simulink model "warp_timer"  (Simulink 7.1)
settings: Solver=ode45  StartTime=0.0  StopTime=1000  RelTol=1e-3
undefined symbols (not defined in the file): gcbh, xlBlockLoadCallback, xlGetSimulinkPeriod
libraries: xbsIndex_r4 x450
(part 1 of 5)
settings Model: Creator=CMC  LastModifiedBy=murphpo
settings DebuggingCC: SaveWithParameterizedLinksMsg=none  SignalResolutionControl=TryResolveAllWithWarning  MultiTaskDSMMsg=warning  MultiTaskCondExecSysMsg=none
settings RTWCC: IncludeERTFirstTime=on
settings GRTTargetCC: TargetFcnLib=ansi_tfl_tmw.mat

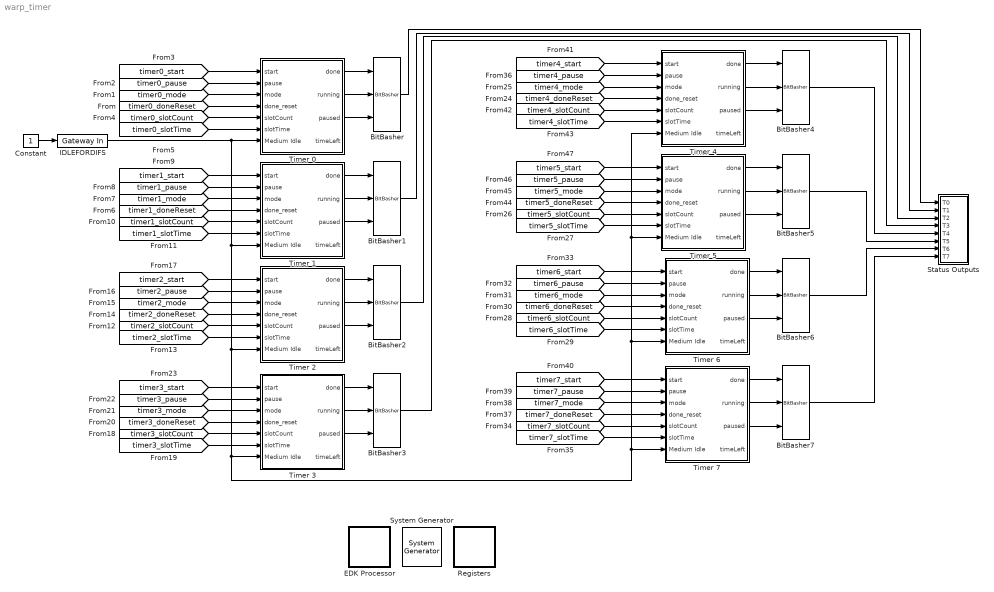
== system warp_timer ==
  " System Generator" : xbsIndex_r4/ System Generator  Tag=genX  SystemSampleTime=-1  xilinxfamily=virtex2p  part=xc2vp70  speed=-6  package=ff1517  synthesis_tool=XST  clock_wrapper=Clock Enables  directory=./pcore_v03  testbench=off  simulink_period=1  sysclk_period=10  dcm_input_clock_period=100  incr_netlist=off  trim_vbits=Everywhere in SubSystem  dbl_ovrd=According to Block Masks  core_generation=According to Block Masks  run_coregen=off  deprecated_control=off  eval_field=0  block_type=sysgen
      settings: block_version=8.2
  BitBasher : xbsIndex_r4/BitBasher  bitexpr=|  display_expr=off  sr_1=1  arith_type1=Unsigned  bin_pt1=0  sr_2=2  arith_type2=Unsigned  bin_pt2=0  sr_3=3  arith_type3=Unsigned  bin_pt3=0  sr_4=4  arith_type4=Unsigned  bin_pt4=0  dbl_ovrd=off  block_type=bitbasher
      | <html><head><meta name="qrichtext" content="1" /><style type="text/css">
      | p, li { white-space: pre-wrap; }
      | </style></head><body style=" font-family:'MS Shell Dlg 2'; font-size:8.25pt; font-weight:400; font-style:normal;">
      | <p style=" margin-top:12px; margin-bottom:12px; margin-left:0px; margin-right:0px; -qt-block-indent:0; text-indent:0px; font-family:'MS Shell Dlg'; font-size:8pt;">Q={1'b0,a,b,c}<br /></p></body></html>
      settings: block_version=10.1.3
  BitBasher1 : xbsIndex_r4/BitBasher  bitexpr=|  display_expr=off  sr_1=1  arith_type1=Unsigned  bin_pt1=0  sr_2=2  arith_type2=Unsigned  bin_pt2=0  sr_3=3  arith_type3=Unsigned  bin_pt3=0  sr_4=4  arith_type4=Unsigned  bin_pt4=0  dbl_ovrd=off  block_type=bitbasher
      | <html><head><meta name="qrichtext" content="1" /><style type="text/css">
      | p, li { white-space: pre-wrap; }
      | </style></head><body style=" font-family:'MS Shell Dlg 2'; font-size:8.25pt; font-weight:400; font-style:normal;">
      | <p style=" margin-top:12px; margin-bottom:12px; margin-left:0px; margin-right:0px; -qt-block-indent:0; text-indent:0px; font-family:'MS Shell Dlg'; font-size:8pt;">Q={1'b0,a,b,c}<br /></p></body></html>
      settings: block_version=10.1.3
  BitBasher2 : xbsIndex_r4/BitBasher  bitexpr=|  display_expr=off  sr_1=1  arith_type1=Unsigned  bin_pt1=0  sr_2=2  arith_type2=Unsigned  bin_pt2=0  sr_3=3  arith_type3=Unsigned  bin_pt3=0  sr_4=4  arith_type4=Unsigned  bin_pt4=0  dbl_ovrd=off  block_type=bitbasher
      | <html><head><meta name="qrichtext" content="1" /><style type="text/css">
      | p, li { white-space: pre-wrap; }
      | </style></head><body style=" font-family:'MS Shell Dlg 2'; font-size:8.25pt; font-weight:400; font-style:normal;">
      | <p style=" margin-top:12px; margin-bottom:12px; margin-left:0px; margin-right:0px; -qt-block-indent:0; text-indent:0px; font-family:'MS Shell Dlg'; font-size:8pt;">Q={1'b0,a,b,c}<br /></p></body></html>
      settings: block_version=10.1.3
  BitBasher3 : xbsIndex_r4/BitBasher  bitexpr=|  display_expr=off  sr_1=1  arith_type1=Unsigned  bin_pt1=0  sr_2=2  arith_type2=Unsigned  bin_pt2=0  sr_3=3  arith_type3=Unsigned  bin_pt3=0  sr_4=4  arith_type4=Unsigned  bin_pt4=0  dbl_ovrd=off  block_type=bitbasher
      | <html><head><meta name="qrichtext" content="1" /><style type="text/css">
      | p, li { white-space: pre-wrap; }
      | </style></head><body style=" font-family:'MS Shell Dlg 2'; font-size:8.25pt; font-weight:400; font-style:normal;">
      | <p style=" margin-top:12px; margin-bottom:12px; margin-left:0px; margin-right:0px; -qt-block-indent:0; text-indent:0px; font-family:'MS Shell Dlg'; font-size:8pt;">Q={1'b0,a,b,c}<br /></p></body></html>
      settings: block_version=10.1.3
  BitBasher4 : xbsIndex_r4/BitBasher  bitexpr=|  display_expr=off  sr_1=1  arith_type1=Unsigned  bin_pt1=0  sr_2=2  arith_type2=Unsigned  bin_pt2=0  sr_3=3  arith_type3=Unsigned  bin_pt3=0  sr_4=4  arith_type4=Unsigned  bin_pt4=0  dbl_ovrd=off  block_type=bitbasher
      | <html><head><meta name="qrichtext" content="1" /><style type="text/css">
      | p, li { white-space: pre-wrap; }
      | </style></head><body style=" font-family:'MS Shell Dlg 2'; font-size:8.25pt; font-weight:400; font-style:normal;">
      | <p style=" margin-top:12px; margin-bottom:12px; margin-left:0px; margin-right:0px; -qt-block-indent:0; text-indent:0px; font-family:'MS Shell Dlg'; font-size:8pt;">Q={1'b0,a,b,c}<br /></p></body></html>
      settings: block_version=10.1.3
  BitBasher5 : xbsIndex_r4/BitBasher  bitexpr=|  display_expr=off  sr_1=1  arith_type1=Unsigned  bin_pt1=0  sr_2=2  arith_type2=Unsigned  bin_pt2=0  sr_3=3  arith_type3=Unsigned  bin_pt3=0  sr_4=4  arith_type4=Unsigned  bin_pt4=0  dbl_ovrd=off  block_type=bitbasher
      | <html><head><meta name="qrichtext" content="1" /><style type="text/css">
      | p, li { white-space: pre-wrap; }
      | </style></head><body style=" font-family:'MS Shell Dlg 2'; font-size:8.25pt; font-weight:400; font-style:normal;">
      | <p style=" margin-top:12px; margin-bottom:12px; margin-left:0px; margin-right:0px; -qt-block-indent:0; text-indent:0px; font-family:'MS Shell Dlg'; font-size:8pt;">Q={1'b0,a,b,c}<br /></p></body></html>
      settings: block_version=10.1.3
  BitBasher6 : xbsIndex_r4/BitBasher  bitexpr=|  display_expr=off  sr_1=1  arith_type1=Unsigned  bin_pt1=0  sr_2=2  arith_type2=Unsigned  bin_pt2=0  sr_3=3  arith_type3=Unsigned  bin_pt3=0  sr_4=4  arith_type4=Unsigned  bin_pt4=0  dbl_ovrd=off  block_type=bitbasher
      | <html><head><meta name="qrichtext" content="1" /><style type="text/css">
      | p, li { white-space: pre-wrap; }
      | </style></head><body style=" font-family:'MS Shell Dlg 2'; font-size:8.25pt; font-weight:400; font-style:normal;">
      | <p style=" margin-top:12px; margin-bottom:12px; margin-left:0px; margin-right:0px; -qt-block-indent:0; text-indent:0px; font-family:'MS Shell Dlg'; font-size:8pt;">Q={1'b0,a,b,c}<br /></p></body></html>
      settings: block_version=10.1.3
  BitBasher7 : xbsIndex_r4/BitBasher  bitexpr=|  display_expr=off  sr_1=1  arith_type1=Unsigned  bin_pt1=0  sr_2=2  arith_type2=Unsigned  bin_pt2=0  sr_3=3  arith_type3=Unsigned  bin_pt3=0  sr_4=4  arith_type4=Unsigned  bin_pt4=0  dbl_ovrd=off  block_type=bitbasher
      | <html><head><meta name="qrichtext" content="1" /><style type="text/css">
      | p, li { white-space: pre-wrap; }
      | </style></head><body style=" font-family:'MS Shell Dlg 2'; font-size:8.25pt; font-weight:400; font-style:normal;">
      | <p style=" margin-top:12px; margin-bottom:12px; margin-left:0px; margin-right:0px; -qt-block-indent:0; text-indent:0px; font-family:'MS Shell Dlg'; font-size:8pt;">Q={1'b0,a,b,c}<br /></p></body></html>
      settings: block_version=10.1.3
  Constant : Constant  OutDataType=sfix(16)  OutScaling=2^0
  EDK Processor : Subsystem  LoadFcn=xlBlockLoadCallback(gcbh);  mask(Xilinx EDK Processor Block){mode=EDK pcore generation, xmp=, MemVisToProc=<qt bgcolor="#FFFFFF"><div><img src="C:\Xilinx\10.1\DSP_Tools\common\bin\..\..\sysgen\data\images\registerplus.gif"> &lt;&lt;timer0_slotCount&gt;&gt;<br></div><div><img src="C:\Xilinx\10.1\DSP_Tools\common\bin\..\..\sysgen\data\images\registerplus.gif"> &lt;&lt;timer1_slotCount&gt;&gt;<br></div><div><img src="C:\Xilinx\10.1\DSP_Tools\common\bin\..\..\sysgen\data\images\registerplus.gif"> &lt;&lt;timer2_slotCount&gt;&gt;<br></div><div><img src="C:\Xilinx\10.1\DSP_Tools\common\bin\..\..\sysgen\data\images\registerplus.gif"> &lt;&lt;timer3_slotCount&gt;&gt;<br></div><div><img src="C:\Xilinx\10.1\DSP_Tools\common\bin\..\..\sysgen\data\images\registerplus.gif"> &lt;&lt;timer4_slotCount&gt;&gt;<br></div><div><img src="C:\Xilinx\10.1\DSP_Tools\common\bin\..\..\sysgen\data\images\registerplus.gif"> &lt;&lt;timer5_slotCount&gt;&gt;<br></div><div><img src="C:\Xilinx\10.1\DSP_Tools\common\bin\..\..\sysgen\data\images\registerplus.gif"> &lt;&lt;timer6_slotCount&gt;&gt;<br></div><div><img src="C:\Xilinx\10.1\DSP_Tools\common\bin\..\..\sysgen\data\images\registerplus.gif"> &lt;&lt;timer7_slotCount&gt;&gt;<br></div><div><img src="C:\Xilinx\10.1\DSP_Tools\common\bin\..\..\sysgen\data\images\registerplus.gif"> &lt;&lt;timer_control&gt;&gt;<br></div><div><img src="C:\Xilinx\10.1\DSP_Tools\common\bin\..\..\sysgen\data\images\registerplus.gif"> &lt;&lt;timer_status&gt;&gt;<br></div><div><img src="C:\Xilinx\10.1\DSP_Tools\common\bin\..\..\sysgen\data\images\registerplus.gif"> &lt;&lt;timers01_slotTime&gt;&gt;<br></div><div><img src="C:\Xilinx\10.1\DSP_Tools\common\bin\..\..\sysgen\data\images\registerplus.gif"> &lt;&lt;timers23_slotTime&gt;&gt;<br></div><div><img src="C:\Xilinx\10.1\DSP_Tools\common\bin\..\..\sysgen\data\images\registerplus.gif"> &lt;&lt;timers45_slotTime&gt;&gt;<br></div><div><img src="C:\Xilinx\10.1\DSP_Tools\common\bin\..\..\sysgen\data\images\registerplus.gif"> &lt;&lt;timers67_slotTime&gt;&gt;<br></div></qt>, AvailableMemories=<empty>, portInterfaceTable={'exposed'=>[],'portdir'=>[],'portname'=>[],'shortname'=>[]}, bus_type_sgadvanced=, bus_type=PLB, baseaddr=0x80000000, baseaddr_lock_sgadvanced=, baseaddr_lock=off, dual_clock_sgadvanced=, dual_clock=off, reg_readback_sgadvanced=, reg_readback=on, ucf_file=, inheritDeviceType_sgadvanced=, inheritDeviceType=off, clock_name=plb, internalPortList={}, resetPolarity=0, memxtable={'mlist'=>['warp_timer/Registers/From Register9','warp_timer/Registers/From Register1','warp_timer/Registers/From Register3','warp_timer/Registers/From Register2','warp_timer/Registers/From Register7','warp_timer/Registers/From Register4','warp_timer/Registers/From Register6','warp_timer/Registers/From Register5','warp_timer/Registers/From Register8','warp_timer/Registers/To Register4','warp_timer/Registers/From Register11','warp_timer/Registers/From Register12','warp_timer/Registers/From Register13','warp_timer/Registers/From Register14'],'mlname'=>['\'timer0_slotCount\'','\'timer1_slotCount\'','\'timer2_slotCount\'','\'timer3_slotCount\'','\'timer4_slotCount\'','\'timer5_slotCount\'','\'timer6_slotCount\'','\'timer7_slotCount\'','\'timer_control\'','\'timer_status\'','\'timers01_slotTime\'','\'timers23_slotTime\'','\'timers45_slotTime\'','\'timers67_slotTime\''],'mlstate'=>[0.00000000000000000,0.00000000000000000,0.00000000000000000,0.00000000000000000,0.00000000000000000,0.00000000000000000,0.00000000000000000,0.00000000000000000,0.00000000000000000,0.00000000000000000,0.00000000000000000,0.00000000000000000,0.00000000000000000,0.00000000000000000]}, procinfo={'xmliface'=>'Xilinx//microblaze//iface.xml'}, memmapdirty=off, blockname=, xpsintstyle=default, has_advanced_control=0, sggui_pos=20,20,383,441, block_type=edkprocessor, block_version=2.5, sg_icon_stat=51,50,-1,-1,white,blue,0,07734,right, sg_mask_display=|, sg_list_contents={'table'=>{'AvailableMemories'=>'popup(<empty>)','userSelections'=>{'AvailableMemories'=>'<empty>'}}}, sg_blockgui_xml=}
      mask sg_mask_display=|
      | fprintf('','COMMENT: begin icon graphics');
      | patch([0 51 51 0 ],[0 0 50 50 ],[0.77 0.82 0.91]);
      | patch([12 4 16 4 12 25 29 33 47 36 25 17 29 17 25 36 47 33 29 25 12 ],[5 13 25 37 45 45 41 45 45 34 45 37 25 13 5 16 5 5 9 5 5 ],[0.98 0.96 0.92]);
      | plot([0 51 51 0 0 ],[0 0 50 50 0 ]);
      | fprintf('','COMMENT: end icon graphics');
      | fprintf('','COMMENT: begin icon text');
      | fprintf('','COMMENT: end icon text');
      mask prompts: mode "Configure Processor for"; xmp "EDK Project"; MemVisToProc ""; AvailableMemories "Available Memories"; portInterfaceTable ""; bus_type_sgadvanced ""; bus_type "Bus Type"; baseaddr "Base Address"; baseaddr_lock_sgadvanced ""; baseaddr_lock "Lock"; dual_clock_sgadvanced ""; dual_clock "Dual Clocks"; reg_readback_sgadvanced ""; reg_readback "Register Read-Back"; ucf_file "Constraint file"; inheritDeviceType_sgadvanced ""; inheritDeviceType "Inherit Device Type"; clock_name ""; internalPortList ""; resetPolarity ""; memxtable ""; procinfo ""; memmapdirty ""; blockname ""; xpsintstyle ""; has_advanced_control ""; sggui_pos ""; block_type ""; block_version ""; sg_icon_stat ""; sg_mask_display ""; sg_list_contents ""; sg_blockgui_xml ""
      mask help: Xilinx EDK Processor
      mask init:
      | try
      |   tmp_gcb = gcb;
      |   tmp_gcbh = gcbh;
      |   if (strcmp('SysGenIndex',get_param(bdroot(tmp_gcbh),'tag')) && ~isempty(regexp(bdroot(tmp_gcb), '^xbs', 'once')))
      |     return;
      |   end;
      |   xlMungeMaskParams;
      | 
      | block_type='edkprocessor';
      |   serialized_declarations = '{,''block_type''=>''String''}';
      |   xledkprocessor_init();
      |   ptable_ = xlblockprep(get_param(tmp_gcb, 'MaskWSVariables'));
      | catch
      |   global dbgsysgen;
      |   if(~isempty(dbgsysgen) && dbgsysgen)
      |     e = regexprep(lasterr, '\n', '\nError: ');
      |     disp(['Error: While running MaskInit code on block ' tmp_gcb ': ' e]);
      |     error(e);
      |   end
      | end
      settings: CopyFcn=xlProcBlockCopyCallback(gcbh);xlBlockMoveCallback(gcbh);  DeleteFcn=xlDestroyGui(gcbh);  ModelCloseFcn=xlDestroyGui(gcbh);  PreSaveFcn=xlBlockPreSaveCallback(gcbh);  PostSaveFcn=xlBlockPostSaveCallback(gcbh);  DestroyFcn=xlDestroyGui(gcbh);  OpenFcn=bh=gcbh;xlProcBlockCallbacks('populatesharedmemorylistbox',bh);xlOpenGui(bh, 'edkprocessor_gui.xml', @xlProcBlockEnablement, @xlProcBlockAction)  CloseFcn=xlDestroyGui(gcbh);  MoveFcn=xlBlockMoveCallback(gcbh);
      mask Help: eval('');xlDoc('-book','sysgen','-topic','EDK_Processor');
      mask StyleString: popup(EDK pcore generation|HDL netlisting),edit,edit,popup(<empty>),edit,edit,popup(PLB|FSL),edit,edit,checkbox,edit,checkbox,edit,checkbox,edit,edit,checkbox,edit,edit,edit,edit,edit,edit,edit,edit,edit,edit,edit,edit,edit,edit,edit,edit
      mask Display:
      | fprintf('','COMMENT: begin icon graphics');
      | patch([0 51 51 0 ],[0 0 50 50 ],[0.77 0.82 0.91]);
      | patch([12 4 16 4 12 25 29 33 47 36 25 17 29 17 25 36 47 33 29 25 12 ],[5 13 25 37 45 45 41 45 45 34 45 37 25 13 5 16 5 5 9 5 5 ],[0.98 0.96 0.92]);
      | plot([0 51 51 0 0 ],[0 0 50 50 0 ]);
      | fprintf('','COMMENT: end icon graphics');
      | fprintf('','COMMENT: begin icon text');
      | disp('');
      | 
      | fprintf('','COMMENT: end icon text');
  IDLEFORDIFS : xbsIndex_r4/Gateway In  arith_type=Unsigned  n_bits=1  bin_pt=0  quantization="Round  (unbiased: +/- Inf)"  overflow=Saturate  period=1  dbl_ovrd=off  timing_constraint=None  locs_specified=off  LOCs={}  block_type=gatewayin
      settings: infoedit="Gateway in block.  Converts inputs of type Simulink integer, double and fixed point to  Xilinx fixed point type.<P><P>Hardware notes:  In hardware these blocks become top level input ports."  block_version=8.2
  Registers : Subsystem
  Status Outputs : Subsystem
  Timer 0 : Subsystem
  Timer 1 : Subsystem
  Timer 2 : Subsystem
  Timer 3 : Subsystem
  Timer 4 : Subsystem
  Timer 5 : Subsystem
  Timer 6 : Subsystem
  Timer 7 : Subsystem
  wires:
  Constant/1 -> IDLEFORDIFS/1
  [timer0_doneReset] -> Timer 0/4(done_reset)
  [timer0_mode] -> Timer 0/3(mode)
  [timer0_pause] -> Timer 0/2(pause)
  [timer0_start] -> Timer 0/1(start)
  [timer0_slotCount] -> Timer 0/5(slotCount)
  [timer0_slotTime] -> Timer 0/6(slotTime)
  [timer1_doneReset] -> Timer 1/4(done_reset)
  [timer1_mode] -> Timer 1/3(mode)
  [timer1_pause] -> Timer 1/2(pause)
  [timer1_start] -> Timer 1/1(start)
  [timer1_slotCount] -> Timer 1/5(slotCount)
  [timer1_slotTime] -> Timer 1/6(slotTime)
  [timer2_doneReset] -> Timer 2/4(done_reset)
  [timer2_mode] -> Timer 2/3(mode)
  [timer2_pause] -> Timer 2/2(pause)
  [timer2_start] -> Timer 2/1(start)
  [timer2_slotCount] -> Timer 2/5(slotCount)
  [timer2_slotTime] -> Timer 2/6(slotTime)
  [timer3_doneReset] -> Timer 3/4(done_reset)
  [timer3_mode] -> Timer 3/3(mode)
  [timer3_pause] -> Timer 3/2(pause)
  [timer3_start] -> Timer 3/1(start)
  [timer3_slotCount] -> Timer 3/5(slotCount)
  [timer3_slotTime] -> Timer 3/6(slotTime)
  [timer4_doneReset] -> Timer 4/4(done_reset)
  [timer4_mode] -> Timer 4/3(mode)
  [timer4_pause] -> Timer 4/2(pause)
  [timer4_start] -> Timer 4/1(start)
  [timer4_slotCount] -> Timer 4/5(slotCount)
  [timer4_slotTime] -> Timer 4/6(slotTime)
  [timer5_doneReset] -> Timer 5/4(done_reset)
  [timer5_mode] -> Timer 5/3(mode)
  [timer5_pause] -> Timer 5/2(pause)
  [timer5_start] -> Timer 5/1(start)
  [timer5_slotCount] -> Timer 5/5(slotCount)
  [timer5_slotTime] -> Timer 5/6(slotTime)
  [timer6_doneReset] -> Timer 6/4(done_reset)
  [timer6_mode] -> Timer 6/3(mode)
  [timer6_pause] -> Timer 6/2(pause)
  [timer6_start] -> Timer 6/1(start)
  [timer6_slotCount] -> Timer 6/5(slotCount)
  [timer6_slotTime] -> Timer 6/6(slotTime)
  [timer7_doneReset] -> Timer 7/4(done_reset)
  [timer7_mode] -> Timer 7/3(mode)
  [timer7_pause] -> Timer 7/2(pause)
  [timer7_start] -> Timer 7/1(start)
  [timer7_slotCount] -> Timer 7/5(slotCount)
  [timer7_slotTime] -> Timer 7/6(slotTime)
  Timer 0/1(done) -> BitBasher/1
  Timer 0/2(running) -> BitBasher/2
  Timer 0/3(paused) -> BitBasher/3
  IDLEFORDIFS/1 -> Timer 0/7(Medium Idle), Timer 4/7(Medium Idle), Timer 5/7(Medium Idle), Timer 6/7(Medium Idle), Timer 7/7(Medium Idle), Timer 3/7(Medium Idle), Timer 2/7(Medium Idle), Timer 1/7(Medium Idle)
  Timer 1/1(done) -> BitBasher1/1
  Timer 1/2(running) -> BitBasher1/2
  Timer 1/3(paused) -> BitBasher1/3
  Timer 2/1(done) -> BitBasher2/1
  Timer 2/2(running) -> BitBasher2/2
  Timer 2/3(paused) -> BitBasher2/3
  Timer 3/1(done) -> BitBasher3/1
  Timer 3/2(running) -> BitBasher3/2
  Timer 3/3(paused) -> BitBasher3/3
  Timer 4/1(done) -> BitBasher4/1
  Timer 4/2(running) -> BitBasher4/2
  Timer 4/3(paused) -> BitBasher4/3
  Timer 5/1(done) -> BitBasher5/1
  Timer 5/2(running) -> BitBasher5/2
  Timer 5/3(paused) -> BitBasher5/3
  Timer 6/1(done) -> BitBasher6/1
  Timer 6/2(running) -> BitBasher6/2
  Timer 6/3(paused) -> BitBasher6/3
  Timer 7/1(done) -> BitBasher7/1
  Timer 7/2(running) -> BitBasher7/2
  Timer 7/3(paused) -> BitBasher7/3
  BitBasher/1 -> Status Outputs/1(T0)
  BitBasher1/1 -> Status Outputs/2(T1)
  BitBasher2/1 -> Status Outputs/3(T2)
  BitBasher3/1 -> Status Outputs/4(T3)
  BitBasher4/1 -> Status Outputs/5(T4)
  BitBasher5/1 -> Status Outputs/6(T5)
  BitBasher6/1 -> Status Outputs/7(T6)
  BitBasher7/1 -> Status Outputs/8(T7)
